simulink model "model"  (R2022b)
settings: Solver=VariableStepAuto  StartTime=0.0  StopTime=15  RelTol=1e-3
libraries: neural x114, simulink x4
(part 4 of 4)

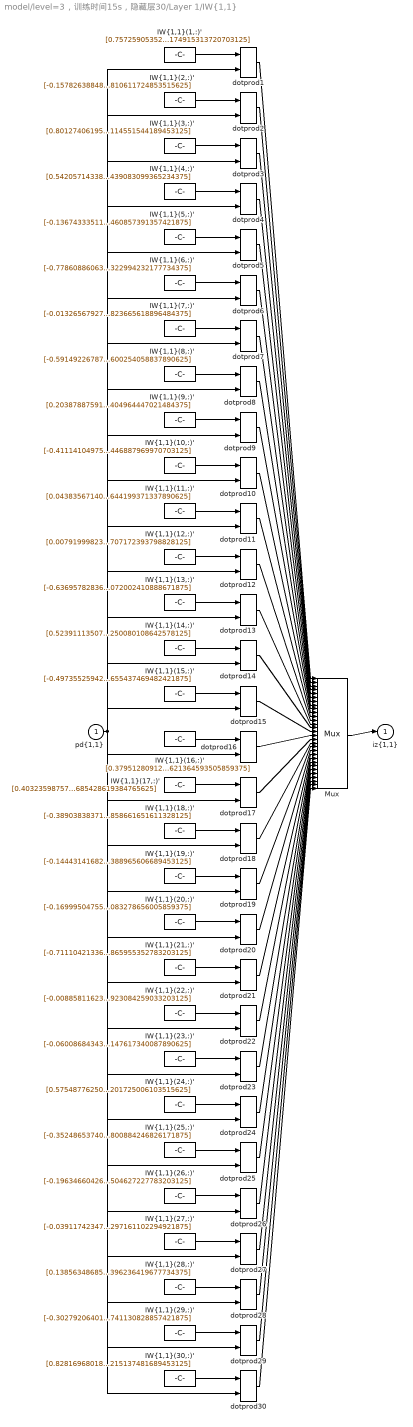
== system model/level=3，训练时间15s，隐藏层30/Layer 1/IW{1,1} ==
  "pd{1,1}" : Inport  PortDimensions=12
      mask Display: e = 0.06;c1 = [120 230 180]/255;c2 = ([120 230 180]+0)/(256+128);c3 = ([120 230 180]+128)/(256+128);patch([0 1 1 0],[0 0 1 1],c1);patch([0 1 1 1-e 1-e 0+e],[0 0 1 1-e 0+e 0+e],c2);patch([0 0 1 1-e 0+e 0+e],[0 1 1 1-e 1-e 0+e],c3);plot([0 1 1 0 0],[0 0 1 1 0]);
  "IW{1,1}(1,:)'" : Constant  Value=[0.75725905352932321168424323332146741449832916259765625;0.395079353687091294755617809641989879310131072998046875;0.284174770009599508835407277729245834052562713623046875;-0.480625127186739498075240817343001253902912139892578125;1.5532866213137079824946340522728860378265380859375;-0.2164618951796444534796393099895794875919818878173828125;1.2456775953176404403421884126146323978900909423828125;-1.10858492845372236246248576208017766475677490234375;0.639442817441132405065218335948884487152099609375;0.293978171890306894109556878902367316186428070068359375;-0.94941996422992291915221585441031493246555328369140625;0.92768764030551065236096519583952613174915313720703125]
      mask Display: e = 0.06;c1 = [120 150 230]/255;c2 = ([120 150 230]+0)/383;c3 = ([120 150 230]+128)/383;patch([0 1 1 0],[0 0 1 1],c1);patch([0 1 1 1-e 1-e 0+e],[0 0 1 1-e 0+e 0+e],c2);patch([0 0 1 1-e 0+e 0+e],[0 1 1 1-e 1-e 0+e],c3);plot([0 1 1 0 0],[0 0 1 1 0]);disp('Weights');
  "IW{1,1}(10,:)'" : Constant  Value=[-0.41114104975904297578637169863213784992694854736328125;0.638123539358462554815787370898760855197906494140625;0.8892656713827828962593002870562486350536346435546875;-0.2296787045340132060733395746865426190197467803955078125;-0.101513006637653280250788156990893185138702392578125;0.1570479389804073921954596926298108883202075958251953125;-0.5212086340938679729362092984956689178943634033203125;0.59304447094252032979255773170734755694866180419921875;0.893787792975378803106423220015130937099456787109375;0.2422359635921390308421763393198489211499691009521484375;0.393771951328514335788355538170435465872287750244140625;-0.0501811485120902400769438145289313979446887969970703125]
      mask Display: e = 0.06;c1 = [120 150 230]/255;c2 = ([120 150 230]+0)/383;c3 = ([120 150 230]+128)/383;patch([0 1 1 0],[0 0 1 1],c1);patch([0 1 1 1-e 1-e 0+e],[0 0 1 1-e 0+e 0+e],c2);patch([0 0 1 1-e 0+e 0+e],[0 1 1 1-e 1-e 0+e],c3);plot([0 1 1 0 0],[0 0 1 1 0]);disp('Weights');
  "IW{1,1}(11,:)'" : Constant  Value=[0.0438356714023393212453783007731544785201549530029296875;0.000584453236434134826282615904347039759159088134765625;0.0234071241969575731534103368858268368057906627655029296875;-0.0146965389691917636127982405014336109161376953125;0.012973200671017141860641430639589088968932628631591796875;-0.0796343916408829011199799197129323147237300872802734375;-0.92626778833588374606478055284242145717144012451171875;0.55553594240003401072414135342114605009555816650390625;0.3147831513142638204527656853315420448780059814453125;0.70814607465412660047832105192355811595916748046875;1.113472027689847099196640556328929960727691650390625;-0.486007529758314016365972065614187158644199371337890625]
      mask Display: e = 0.06;c1 = [120 150 230]/255;c2 = ([120 150 230]+0)/383;c3 = ([120 150 230]+128)/383;patch([0 1 1 0],[0 0 1 1],c1);patch([0 1 1 1-e 1-e 0+e],[0 0 1 1-e 0+e 0+e],c2);patch([0 0 1 1-e 0+e 0+e],[0 1 1 1-e 1-e 0+e],c3);plot([0 1 1 0 0],[0 0 1 1 0]);disp('Weights');
  "IW{1,1}(12,:)'" : Constant  Value=[0.00791999823281246649597786557706058374606072902679443359375;-0.000416308322128628783588555339889580864110030233860015869140625;0.007136286944569004107863374741782536148093640804290771484375;-0.004813165301803152239246141874673412530682981014251708984375;0.004455198856121612462077852256925325491465628147125244140625;-0.0158514264036779990718617483480556984432041645050048828125;0.76581982923121127981858080602250993251800537109375;1.082796206543517048004332536947913467884063720703125;1.0764809157713461917893482677754946053028106689453125;0.75575388653398001270744543944601900875568389892578125;-0.694644687537094629448120031156577169895172119140625;-0.7383832671373753431254272072692401707172393798828125]
      mask Display: e = 0.06;c1 = [120 150 230]/255;c2 = ([120 150 230]+0)/383;c3 = ([120 150 230]+128)/383;patch([0 1 1 0],[0 0 1 1],c1);patch([0 1 1 1-e 1-e 0+e],[0 0 1 1-e 0+e 0+e],c2);patch([0 0 1 1-e 0+e 0+e],[0 1 1 1-e 1-e 0+e],c3);plot([0 1 1 0 0],[0 0 1 1 0]);disp('Weights');
  "IW{1,1}(13,:)'" : Constant  Value=[-0.63695782836304826179940619113040156662464141845703125;0.629096052803664207431211252696812152862548828125;0.323311497459243757379709904853370971977710723876953125;-0.10905608847097224278765992266926332376897335052490234375;0.00182196457625318874833098004017983839730732142925262451171875;-0.40021595696852230172879671954433433711528778076171875;-0.58507556697968521319808132830075919628143310546875;-0.1289161268611479782553175255088717676699161529541015625;0.70346509838735793440633869977318681776523590087890625;0.758628536034963385503715471713803708553314208984375;1.0820696215042822085905527274007908999919891357421875;0.66331696609620649507377265763352625072002410888671875]
      mask Display: e = 0.06;c1 = [120 150 230]/255;c2 = ([120 150 230]+0)/383;c3 = ([120 150 230]+128)/383;patch([0 1 1 0],[0 0 1 1],c1);patch([0 1 1 1-e 1-e 0+e],[0 0 1 1-e 0+e 0+e],c2);patch([0 0 1 1-e 0+e 0+e],[0 1 1 1-e 1-e 0+e],c3);plot([0 1 1 0 0],[0 0 1 1 0]);disp('Weights');
  "IW{1,1}(14,:)'" : Constant  Value=[0.52391113507237629942636658597621135413646697998046875;0.748442776635961148912201679195277392864227294921875;-0.5994868462670253084212390604079701006412506103515625;-0.407014205676378637566159568450530059635639190673828125;0.6801681371389649566339130615233443677425384521484375;-0.1601777419913940903040128205248038284480571746826171875;0.591124691698642124038087786175310611724853515625;-0.60466411573088463260461367099196650087833404541015625;-0.1698340507383852282519143273020745255053043365478515625;0.322498129489360685351329038894618861377239227294921875;-0.0207917527819724036464155147996279993094503879547119140625;0.45280346894891909670377572183497250080108642578125]
      mask Display: e = 0.06;c1 = [120 150 230]/255;c2 = ([120 150 230]+0)/383;c3 = ([120 150 230]+128)/383;patch([0 1 1 0],[0 0 1 1],c1);patch([0 1 1 1-e 1-e 0+e],[0 0 1 1-e 0+e 0+e],c2);patch([0 0 1 1-e 0+e 0+e],[0 1 1 1-e 1-e 0+e],c3);plot([0 1 1 0 0],[0 0 1 1 0]);disp('Weights');
  "IW{1,1}(15,:)'" : Constant  Value=[-0.4973552594221628542214830304146744310855865478515625;-0.57340079597389592702683103198069147765636444091796875;0.2404892307980655286048232710527372546494007110595703125;0.14602880061020651059067176902317441999912261962890625;-0.4128068227448673521706723477109335362911224365234375;-0.449657532232850043474314816194237209856510162353515625;-0.437774623382925665016074390223366208374500274658203125;-0.0506924454175674277234264764047111384570598602294921875;0.03919016699132422953955057209896040149033069610595703125;-0.318569485200799917823388796023209579288959503173828125;-1.0445535535771595103682329863659106194972991943359375;1.5582165788630042424500743436510674655437469482421875]
      mask Display: e = 0.06;c1 = [120 150 230]/255;c2 = ([120 150 230]+0)/383;c3 = ([120 150 230]+128)/383;patch([0 1 1 0],[0 0 1 1],c1);patch([0 1 1 1-e 1-e 0+e],[0 0 1 1-e 0+e 0+e],c2);patch([0 0 1 1-e 0+e 0+e],[0 1 1 1-e 1-e 0+e],c3);plot([0 1 1 0 0],[0 0 1 1 0]);disp('Weights');
  "IW{1,1}(16,:)'" : Constant  Value=[0.379512809123591920990037351657520048320293426513671875;0.65302219172945097369620270910672843456268310546875;0.2093694388414068241477394849425763823091983795166015625;0.53901943330297819034768735946272499859333038330078125;0.33835271552903611880225298591540195047855377197265625;0.474312833179603376976274375920183956623077392578125;0.2112993037316006350589958628916065208613872528076171875;-0.24506554704123661991843619034625589847564697265625;0.54971876255830476321051492050173692405223846435546875;1.2430077042784175578304939335794188082218170166015625;0.4314133185581263685293151866062544286251068115234375;0.7864615366629035264622871181927621364593505859375]
      mask Display: e = 0.06;c1 = [120 150 230]/255;c2 = ([120 150 230]+0)/383;c3 = ([120 150 230]+128)/383;patch([0 1 1 0],[0 0 1 1],c1);patch([0 1 1 1-e 1-e 0+e],[0 0 1 1-e 0+e 0+e],c2);patch([0 0 1 1-e 0+e 0+e],[0 1 1 1-e 1-e 0+e],c3);plot([0 1 1 0 0],[0 0 1 1 0]);disp('Weights');
  "IW{1,1}(17,:)'" : Constant  Value=[0.403235987579470656072544443304650485515594482421875;-0.1362114449718113406984087987439124844968318939208984375;-0.1822965898937449480410322166790137998759746551513671875;-0.489926907426365965125825141512905247509479522705078125;-0.32566431987358368527196716968319378793239593505859375;-0.1290782481439954054724950083254952915012836456298828125;-0.98752010009051549577208106711623258888721466064453125;-0.155169136490018344520791515606106258928775787353515625;0.3678391748322893395339860944659449160099029541015625;-0.51093268181998385824016395417856983840465545654296875;-0.56491649164861390541858554570353589951992034912109375;-0.488184828165648898590234239236451685428619384765625]
      mask Display: e = 0.06;c1 = [120 150 230]/255;c2 = ([120 150 230]+0)/383;c3 = ([120 150 230]+128)/383;patch([0 1 1 0],[0 0 1 1],c1);patch([0 1 1 1-e 1-e 0+e],[0 0 1 1-e 0+e 0+e],c2);patch([0 0 1 1-e 0+e 0+e],[0 1 1 1-e 1-e 0+e],c3);plot([0 1 1 0 0],[0 0 1 1 0]);disp('Weights');
  "IW{1,1}(18,:)'" : Constant  Value=[-0.389038383711070634429773917872807942330837249755859375;0.420319497494296978601369119132868945598602294921875;-0.351918184281379831102043453938676975667476654052734375;0.04480775966626733552988781639214721508324146270751953125;0.1814472958334386876178001557491370476782321929931640625;-0.21879895422863615550568283651955425739288330078125;-0.358468282492263312644098505188594572246074676513671875;0.196359806412406523445923767212661914527416229248046875;0.6642308737386832806492975578294135630130767822265625;0.1549977942349778647912472706593689508736133575439453125;-0.7313716204282820765314454547478817403316497802734375;-0.63985926564271977667885948903858661651611328125]
      mask Display: e = 0.06;c1 = [120 150 230]/255;c2 = ([120 150 230]+0)/383;c3 = ([120 150 230]+128)/383;patch([0 1 1 0],[0 0 1 1],c1);patch([0 1 1 1-e 1-e 0+e],[0 0 1 1-e 0+e 0+e],c2);patch([0 0 1 1-e 0+e 0+e],[0 1 1 1-e 1-e 0+e],c3);plot([0 1 1 0 0],[0 0 1 1 0]);disp('Weights');
  "IW{1,1}(19,:)'" : Constant  Value=[-0.144431416823362857027035488499677740037441253662109375;-0.999290810935264062209171243011951446533203125;-0.6064844945590530667089979033335112035274505615234375;0.307419146554513245117590258814743719995021820068359375;0.51981343569719717923049984165118075907230377197265625;-1.022888772059110440437734723673202097415924072265625;0.2678751539195631803380592828034423291683197021484375;0.08165050161507102222113729794727987609803676605224609375;0.5316342490032222034557207734906114637851715087890625;-0.079997224310751458009605130428099073469638824462890625;-0.99517161158581834978775759736890904605388641357421875;0.07310073594289434595339116640388965606689453125]
      mask Display: e = 0.06;c1 = [120 150 230]/255;c2 = ([120 150 230]+0)/383;c3 = ([120 150 230]+128)/383;patch([0 1 1 0],[0 0 1 1],c1);patch([0 1 1 1-e 1-e 0+e],[0 0 1 1-e 0+e 0+e],c2);patch([0 0 1 1-e 0+e 0+e],[0 1 1 1-e 1-e 0+e],c3);plot([0 1 1 0 0],[0 0 1 1 0]);disp('Weights');
  "IW{1,1}(2,:)'" : Constant  Value=[-0.1578263884876335010343240128349862061440944671630859375;-0.458760873909689281813228944884031079709529876708984375;-0.305984546669152146503023459445103071630001068115234375;0.58581045035913437146746218786574900150299072265625;-0.047317706603537811049786654393756180070340633392333984375;0.42130501846705092905409628656343556940555572509765625;-0.57844534526135105156896543121547438204288482666015625;0.61224458343678289651279555982910096645355224609375;-0.9387301596170674056196503443061374127864837646484375;-0.044427698494935496942304098411113955080509185791015625;0.32438244619906420052046769342268817126750946044921875;-0.2192552159109796561242688994752825237810611724853515625]
      mask Display: e = 0.06;c1 = [120 150 230]/255;c2 = ([120 150 230]+0)/383;c3 = ([120 150 230]+128)/383;patch([0 1 1 0],[0 0 1 1],c1);patch([0 1 1 1-e 1-e 0+e],[0 0 1 1-e 0+e 0+e],c2);patch([0 0 1 1-e 0+e 0+e],[0 1 1 1-e 1-e 0+e],c3);plot([0 1 1 0 0],[0 0 1 1 0]);disp('Weights');
  "IW{1,1}(20,:)'" : Constant  Value=[-0.16999504755105177000729099745512939989566802978515625;-0.2307373712636667517639210700508556328713893890380859375;0.0887272338162874152356351942216861061751842498779296875;-0.30921237886105645831236188314505852758884429931640625;-0.085253712142476512081401551768067292869091033935546875;0.30098321919776793720302521251142024993896484375;1.0702575958242466214187516015954315662384033203125;0.31550484693018121529206609920947812497615814208984375;0.3615258196366675225164044604753144085407257080078125;-0.00158854198173050890734170348395082328352145850658416748046875;-0.423955871671502670938735946037922985851764678955078125;0.83912806509913406838307992074987851083278656005859375]
      mask Display: e = 0.06;c1 = [120 150 230]/255;c2 = ([120 150 230]+0)/383;c3 = ([120 150 230]+128)/383;patch([0 1 1 0],[0 0 1 1],c1);patch([0 1 1 1-e 1-e 0+e],[0 0 1 1-e 0+e 0+e],c2);patch([0 0 1 1-e 0+e 0+e],[0 1 1 1-e 1-e 0+e],c3);plot([0 1 1 0 0],[0 0 1 1 0]);disp('Weights');
  "IW{1,1}(21,:)'" : Constant  Value=[-0.7111042133619023264401448614080436527729034423828125;-0.6247844908542052877464811899699270725250244140625;-0.411286070103796086439018608871265314519405364990234375;0.50546004210985107096831825401750393211841583251953125;-0.017630168364032729189094794719494529999792575836181640625;0.465225631858145416419603179747355170547962188720703125;-0.489030347200887283154457918499247170984745025634765625;0.34997890668509945566455598964239470660686492919921875;1.2310428148694978478516759423655457794666290283203125;-0.236218929215159134660240169978351332247257232666015625;0.6064418661417680933567453394061885774135589599609375;0.539387507602196780709391532582230865955352783203125]
      mask Display: e = 0.06;c1 = [120 150 230]/255;c2 = ([120 150 230]+0)/383;c3 = ([120 150 230]+128)/383;patch([0 1 1 0],[0 0 1 1],c1);patch([0 1 1 1-e 1-e 0+e],[0 0 1 1-e 0+e 0+e],c2);patch([0 0 1 1-e 0+e 0+e],[0 1 1 1-e 1-e 0+e],c3);plot([0 1 1 0 0],[0 0 1 1 0]);disp('Weights');
  "IW{1,1}(22,:)'" : Constant  Value=[-0.00885811623799481924479426453444830258376896381378173828125;0.001129260518233908029694934072040268802084028720855712890625;-0.00783442931556284187510907912610491621308028697967529296875;0.0064317418415292711142416948177924496121704578399658203125;-0.005060795156085261779776995894053470692597329616546630859375;0.0202300155601852875431045930554319056682288646697998046875;0.1497182692598838238406955269965692423284053802490234375;0.62596589744369257601874778629280626773834228515625;-0.498198984154921309386310213085380382835865020751953125;-1.032780371682340270211852839565835893154144287109375;-0.01657765371532306242219334535548114217817783355712890625;0.43974659987180342302082181049627251923084259033203125]
      mask Display: e = 0.06;c1 = [120 150 230]/255;c2 = ([120 150 230]+0)/383;c3 = ([120 150 230]+128)/383;patch([0 1 1 0],[0 0 1 1],c1);patch([0 1 1 1-e 1-e 0+e],[0 0 1 1-e 0+e 0+e],c2);patch([0 0 1 1-e 0+e 0+e],[0 1 1 1-e 1-e 0+e],c3);plot([0 1 1 0 0],[0 0 1 1 0]);disp('Weights');
  "IW{1,1}(23,:)'" : Constant  Value=[-0.06008684343657157145290881317123421467840671539306640625;0.01367215496164737344175765798581778653897345066070556640625;-0.038969270528510270568123274870231398381292819976806640625;0.022194456059804433534221601576064131222665309906005859375;-0.01341113093208178529136542778132934472523629665374755859375;0.09922945233834022660257545567219494841992855072021484375;0.65314267254930225004017074752482585608959197998046875;-0.45144024693216289190189627333893440663814544677734375;-0.94194454619317913302012357235071249306201934814453125;-0.2252271298497275087147073691085097379982471466064453125;-0.205636323968237999526564863117528147995471954345703125;-0.344140829990361718504487953396164812147617340087890625]
      mask Display: e = 0.06;c1 = [120 150 230]/255;c2 = ([120 150 230]+0)/383;c3 = ([120 150 230]+128)/383;patch([0 1 1 0],[0 0 1 1],c1);patch([0 1 1 1-e 1-e 0+e],[0 0 1 1-e 0+e 0+e],c2);patch([0 0 1 1-e 0+e 0+e],[0 1 1 1-e 1-e 0+e],c3);plot([0 1 1 0 0],[0 0 1 1 0]);disp('Weights');
  "IW{1,1}(24,:)'" : Constant  Value=[0.57548776250792565978287029793136753141880035400390625;-0.45795778096452643968206075442139990627765655517578125;-0.38607748218673354489993698734906502068042755126953125;0.4916252004689363186429318375303409993648529052734375;0.2406619633258665624797600912643247283995151519775390625;-0.8457958795838391719001947421929799020290374755859375;0.372315286864318528703421407044515945017337799072265625;0.72529018681633028453603628804557956755161285400390625;0.35433543342820394972392250565462745726108551025390625;-0.41379597149052071980435130171827040612697601318359375;-0.1366403163625886374443751947183045558631420135498046875;-1.3857644267861051190493526519276201725006103515625]
      mask Display: e = 0.06;c1 = [120 150 230]/255;c2 = ([120 150 230]+0)/383;c3 = ([120 150 230]+128)/383;patch([0 1 1 0],[0 0 1 1],c1);patch([0 1 1 1-e 1-e 0+e],[0 0 1 1-e 0+e 0+e],c2);patch([0 0 1 1-e 0+e 0+e],[0 1 1 1-e 1-e 0+e],c3);plot([0 1 1 0 0],[0 0 1 1 0]);disp('Weights');
  "IW{1,1}(25,:)'" : Constant  Value=[-0.352486537409815336996388168699922971427440643310546875;0.414043250901561632471015172995976172387599945068359375;-0.68290105169643278149038678748183883726596832275390625;-0.96276684869885087447727300968836061656475067138671875;0.5424616924357665848077658665715716779232025146484375;0.1577350356187188495926676523595233447849750518798828125;0.418964763852672394950360512666520662605762481689453125;0.457891452988993197248390742970514111220836639404296875;0.08332747072123615483807412829264649190008640289306640625;0.65158691952563863036829161501373164355754852294921875;-0.76207838543505646011766430092393420636653900146484375;-1.0240547489832934058284763523261062800884246826171875]
      mask Display: e = 0.06;c1 = [120 150 230]/255;c2 = ([120 150 230]+0)/383;c3 = ([120 150 230]+128)/383;patch([0 1 1 0],[0 0 1 1],c1);patch([0 1 1 1-e 1-e 0+e],[0 0 1 1-e 0+e 0+e],c2);patch([0 0 1 1-e 0+e 0+e],[0 1 1 1-e 1-e 0+e],c3);plot([0 1 1 0 0],[0 0 1 1 0]);disp('Weights');
  "IW{1,1}(26,:)'" : Constant  Value=[-0.1963466042652797505230211072557722218334674835205078125;-0.27192840713707522315445430649560876190662384033203125;0.182210292232644344156966553782694973051548004150390625;-0.447224059368448223494851845316588878631591796875;0.1576605364208199799858078904435387812554836273193359375;0.78926919129368589000961264900979585945606231689453125;-1.2972634275407397552726251888088881969451904296875;-0.04020699212536023303687926500060711987316608428955078125;0.487034869518653767972438117794808931648731231689453125;0.6254254757920250096248082627425901591777801513671875;-0.26065496508075458592657014378346502780914306640625;-1.0041097040721507216431973574799485504627227783203125]
      mask Display: e = 0.06;c1 = [120 150 230]/255;c2 = ([120 150 230]+0)/383;c3 = ([120 150 230]+128)/383;patch([0 1 1 0],[0 0 1 1],c1);patch([0 1 1 1-e 1-e 0+e],[0 0 1 1-e 0+e 0+e],c2);patch([0 0 1 1-e 0+e 0+e],[0 1 1 1-e 1-e 0+e],c3);plot([0 1 1 0 0],[0 0 1 1 0]);disp('Weights');
  "IW{1,1}(27,:)'" : Constant  Value=[-0.03911742347526304952598508180017233826220035552978515625;0.494928256667255705991692593670450150966644287109375;-0.461046038716595718565116612808196805417537689208984375;-0.475821016979017408221608320673112757503986358642578125;0.1715992837547896388006307688556262291967868804931640625;0.441321179942003372076442246907390654087066650390625;0.07770246050736133447411901897794450633227825164794921875;-0.7399663724277554255337463473551906645298004150390625;-0.054265638891030233692536199896494508720934391021728515625;-0.84771877074509627281173607116215862333774566650390625;0.491481003922895232083334349226788617670536041259765625;0.362234471234642974035722318149055354297161102294921875]
      mask Display: e = 0.06;c1 = [120 150 230]/255;c2 = ([120 150 230]+0)/383;c3 = ([120 150 230]+128)/383;patch([0 1 1 0],[0 0 1 1],c1);patch([0 1 1 1-e 1-e 0+e],[0 0 1 1-e 0+e 0+e],c2);patch([0 0 1 1-e 0+e 0+e],[0 1 1 1-e 1-e 0+e],c3);plot([0 1 1 0 0],[0 0 1 1 0]);disp('Weights');
  "IW{1,1}(28,:)'" : Constant  Value=[0.1385634868509460215779682812353712506592273712158203125;0.1279689227168545329060833637413452379405498504638671875;-0.11494143852620981871570648991109919734299182891845703125;0.20340717598419566503054056738619692623615264892578125;0.08727794408846646645461220259676338173449039459228515625;-0.283290172800760908788930692026042379438877105712890625;0.160823631436447567200076491644722409546375274658203125;-0.320376770185884340857995766782551072537899017333984375;0.737629304081023118300208807340823113918304443359375;0.63998442620449991213860130301327444612979888916015625;-0.92223956712347021635878263623453676700592041015625;-0.49126791669202185541820426806225441396236419677734375]
      mask Display: e = 0.06;c1 = [120 150 230]/255;c2 = ([120 150 230]+0)/383;c3 = ([120 150 230]+128)/383;patch([0 1 1 0],[0 0 1 1],c1);patch([0 1 1 1-e 1-e 0+e],[0 0 1 1-e 0+e 0+e],c2);patch([0 0 1 1-e 0+e 0+e],[0 1 1 1-e 1-e 0+e],c3);plot([0 1 1 0 0],[0 0 1 1 0]);disp('Weights');
  "IW{1,1}(29,:)'" : Constant  Value=[-0.30279206401474556553665706815081648528575897216796875;-0.412469215746285422508066176305874250829219818115234375;-0.432449526865937350361690505451406352221965789794921875;-0.56925500452449007138255865356768481433391571044921875;-0.059863877680234288403138265266534290276467800140380859375;0.58350248883230182439518785031395964324474334716796875;-0.669606012141286566219378073583357036113739013671875;-0.97190522552113300935872075569932349026203155517578125;-0.63078228616375719983722092365496791899204254150390625;0.70291498121659945486072729181614704430103302001953125;-0.614409800146754836447371417307294905185699462890625;0.125911678355542289153845558757893741130828857421875]
      mask Display: e = 0.06;c1 = [120 150 230]/255;c2 = ([120 150 230]+0)/383;c3 = ([120 150 230]+128)/383;patch([0 1 1 0],[0 0 1 1],c1);patch([0 1 1 1-e 1-e 0+e],[0 0 1 1-e 0+e 0+e],c2);patch([0 0 1 1-e 0+e 0+e],[0 1 1 1-e 1-e 0+e],c3);plot([0 1 1 0 0],[0 0 1 1 0]);disp('Weights');
  "IW{1,1}(3,:)'" : Constant  Value=[0.8012740619552223275690039372420869767665863037109375;-0.7633715123897300003363852738402783870697021484375;-0.465703691458938251468424596168915741145610809326171875;0.03666851099753165588168712929473258554935455322265625;-0.2460643798862774678237741454722709022462368011474609375;-0.162877941160530503861281204081024043262004852294921875;0.545551433681740416403727067518047988414764404296875;0.94833875724121974304381410547648556530475616455078125;0.52080467915547845603185805885004810988903045654296875;0.2174677890345051156639755163269001059234142303466796875;-1.068422894633431763367070743697695434093475341796875;0.334523901695165382097485462509212084114551544189453125]
      mask Display: e = 0.06;c1 = [120 150 230]/255;c2 = ([120 150 230]+0)/383;c3 = ([120 150 230]+128)/383;patch([0 1 1 0],[0 0 1 1],c1);patch([0 1 1 1-e 1-e 0+e],[0 0 1 1-e 0+e 0+e],c2);patch([0 0 1 1-e 0+e 0+e],[0 1 1 1-e 1-e 0+e],c3);plot([0 1 1 0 0],[0 0 1 1 0]);disp('Weights');
  "IW{1,1}(30,:)'" : Constant  Value=[0.82816968018509573568053383496589958667755126953125;0.9201804860082936077247950379387475550174713134765625;0.0955833140605594488992124979631626047194004058837890625;0.572857804385419999704254223615862429141998291015625;0.5228942181369493624742972315289080142974853515625;0.7683928307468963492254943048465065658092498779296875;0.583383677465624916891329121426679193973541259765625;0.288500493038154781633153334041708149015903472900390625;0.482505378597943235252643034982611425220966339111328125;0.0061240261079962728107961567047823336906731128692626953125;0.9410942585011101702008318170555867254734039306640625;0.148252366927580869759850656919297762215137481689453125]
      mask Display: e = 0.06;c1 = [120 150 230]/255;c2 = ([120 150 230]+0)/383;c3 = ([120 150 230]+128)/383;patch([0 1 1 0],[0 0 1 1],c1);patch([0 1 1 1-e 1-e 0+e],[0 0 1 1-e 0+e 0+e],c2);patch([0 0 1 1-e 0+e 0+e],[0 1 1 1-e 1-e 0+e],c3);plot([0 1 1 0 0],[0 0 1 1 0]);disp('Weights');
  "IW{1,1}(4,:)'" : Constant  Value=[0.5420571433834135977036794429295696318149566650390625;-0.1474756847674350279664423624126357026398181915283203125;-0.365439776403620630862434381924686022102832794189453125;0.7077497085807333832008225726895034313201904296875;1.0487685096710299692546186633990146219730377197265625;-0.35569914837861171807986693238490261137485504150390625;-0.552399027313476675971060103620402514934539794921875;-0.2147081738626088476262765425417455844581127166748046875;0.59383018589869662751112855403334833681583404541015625;0.85026968267060476502905430606915615499019622802734375;-0.0192523512445413429172713648540593567304313182830810546875;0.0287311566380798986963807095662559731863439083099365234375]
      mask Display: e = 0.06;c1 = [120 150 230]/255;c2 = ([120 150 230]+0)/383;c3 = ([120 150 230]+128)/383;patch([0 1 1 0],[0 0 1 1],c1);patch([0 1 1 1-e 1-e 0+e],[0 0 1 1-e 0+e 0+e],c2);patch([0 0 1 1-e 0+e 0+e],[0 1 1 1-e 1-e 0+e],c3);plot([0 1 1 0 0],[0 0 1 1 0]);disp('Weights');
  "IW{1,1}(5,:)'" : Constant  Value=[-0.1367433351147859521557137441050144843757152557373046875;-0.060410553566593007401852588600377202965319156646728515625;0.10997569628914076467207650011914665810763835906982421875;-0.004579366895770255359299216735280424472875893115997314453125;0.290226317818353229949224214578862302005290985107421875;0.3481346428669691572821420777472667396068572998046875;0.496980705700768410348899806194822303950786590576171875;-0.4878505757218436489353052820661105215549468994140625;-0.292932542648377147731508785000187344849109649658203125;-0.64064664844808183463698014747933484613895416259765625;-1.1368564158628868820954949114820919930934906005859375;0.52022106413102242594703739086980931460857391357421875]
      mask Display: e = 0.06;c1 = [120 150 230]/255;c2 = ([120 150 230]+0)/383;c3 = ([120 150 230]+128)/383;patch([0 1 1 0],[0 0 1 1],c1);patch([0 1 1 1-e 1-e 0+e],[0 0 1 1-e 0+e 0+e],c2);patch([0 0 1 1-e 0+e 0+e],[0 1 1 1-e 1-e 0+e],c3);plot([0 1 1 0 0],[0 0 1 1 0]);disp('Weights');
  "IW{1,1}(6,:)'" : Constant  Value=[-0.7786088606380554555386197534971870481967926025390625;1.0631936368359100608671496956958435475826263427734375;0.7410329806340187897006899220286868512630462646484375;0.48671035274339813359034678796888329088687896728515625;-0.16755322222335333748333141556940972805023193359375;-1.052994665323438550075252351234667003154754638671875;0.55960633469295950614963430780335329473018646240234375;1.0334851014872141750089440392912365496158599853515625;-0.18471697837201939140783224502229131758213043212890625;0.060399284747913152548992599122357205487787723541259765625;-0.33699098710674346701665626824251376092433929443359375;-0.231368893896155947143000730648054741322994232177734375]
      mask Display: e = 0.06;c1 = [120 150 230]/255;c2 = ([120 150 230]+0)/383;c3 = ([120 150 230]+128)/383;patch([0 1 1 0],[0 0 1 1],c1);patch([0 1 1 1-e 1-e 0+e],[0 0 1 1-e 0+e 0+e],c2);patch([0 0 1 1-e 0+e 0+e],[0 1 1 1-e 1-e 0+e],c3);plot([0 1 1 0 0],[0 0 1 1 0]);disp('Weights');
  "IW{1,1}(7,:)'" : Constant  Value=[-0.0132656792799620941447624744569111499004065990447998046875;-0.00109241586046383300744044841934510259306989610195159912109375;-0.0161138187616071508478921003870709682814776897430419921875;0.012457151836826003965530418327034567482769489288330078125;-0.00814316138631742368614307991947498521767556667327880859375;0.030624545708644874963955118118974496610462665557861328125;-0.55159842387257762563734786454006098210811614990234375;0.35132025843639447248989426952903158962726593017578125;0.6901610288367854284530267250374890863895416259765625;0.08295849322685887317074815427986322902143001556396484375;-0.65282286739034589562180599386920221149921417236328125;-0.430855205660852946802918950197636149823665618896484375]
      mask Display: e = 0.06;c1 = [120 150 230]/255;c2 = ([120 150 230]+0)/383;c3 = ([120 150 230]+128)/383;patch([0 1 1 0],[0 0 1 1],c1);patch([0 1 1 1-e 1-e 0+e],[0 0 1 1-e 0+e 0+e],c2);patch([0 0 1 1-e 0+e 0+e],[0 1 1 1-e 1-e 0+e],c3);plot([0 1 1 0 0],[0 0 1 1 0]);disp('Weights');
  "IW{1,1}(8,:)'" : Constant  Value=[-0.5914922678721143967095486004836857318878173828125;0.1542183272763184564979610513546504080295562744140625;-0.4595809487012003646810853751958347856998443603515625;-0.1405069870888906724548661486551281996071338653564453125;-0.5823603127411878244146237193490378558635711669921875;0.602835725793367860347871101112104952335357666015625;-0.75253374870000400154168573862989433109760284423828125;-0.463913367975307633361836678886902518570423126220703125;0.8908048921767466321597339629079215228557586669921875;-0.5813444755329033597490706597454845905303955078125;-0.83879002630134891216329151575337164103984832763671875;0.202672827905192642905518596307956613600254058837890625]
      mask Display: e = 0.06;c1 = [120 150 230]/255;c2 = ([120 150 230]+0)/383;c3 = ([120 150 230]+128)/383;patch([0 1 1 0],[0 0 1 1],c1);patch([0 1 1 1-e 1-e 0+e],[0 0 1 1-e 0+e 0+e],c2);patch([0 0 1 1-e 0+e 0+e],[0 1 1 1-e 1-e 0+e],c3);plot([0 1 1 0 0],[0 0 1 1 0]);disp('Weights');
  "IW{1,1}(9,:)'" : Constant  Value=[0.2038788759172467102143144757064874283969402313232421875;0.9175756806186854408480257916380651295185089111328125;0.43837184921573857376841942823375575244426727294921875;0.63113247497029700827653186934185214340686798095703125;0.5098618110055361807297913401271216571331024169921875;-0.061984745820637253410634315287097706459462642669677734375;-0.67027740871008634204741838402696885168552398681640625;0.93645585298595179768454954682965762913227081298828125;-0.1298098262110914113964810212564771063625812530517578125;0.34103186031137600053853020654059946537017822265625;-0.299637042573452860860783175667165778577327728271484375;0.36984091827835940957669436102150939404964447021484375]
      mask Display: e = 0.06;c1 = [120 150 230]/255;c2 = ([120 150 230]+0)/383;c3 = ([120 150 230]+128)/383;patch([0 1 1 0],[0 0 1 1],c1);patch([0 1 1 1-e 1-e 0+e],[0 0 1 1-e 0+e 0+e],c2);patch([0 0 1 1-e 0+e 0+e],[0 1 1 1-e 1-e 0+e],c3);plot([0 1 1 0 0],[0 0 1 1 0]);disp('Weights');
  Mux : Mux  Inputs=30
      mask Display: e = 0.06;c1 = [120 150 230]/255;c2 = ([120 150 230]+0)/383;c3 = ([120 150 230]+128)/383;patch([0 1 1 0],[0 0 1 1],c1);patch([0 1 1 1-e 1-e 0+e],[0 0 1 1-e 0+e 0+e],c2);patch([0 0 1 1-e 0+e 0+e],[0 1 1 1-e 1-e 0+e],c3);plot([0 1 1 0 0],[0 0 1 1 0]);disp('Mux');
  dotprod{1..30} (30 alike) : neural/Weight Functions/dotprod
  "iz{1,1}" : Outport
      mask Display: e = 0.06;c1 = [120 230 180]/255;c2 = ([120 230 180]+0)/(256+128);c3 = ([120 230 180]+128)/(256+128);patch([0 1 1 0],[0 0 1 1],c1);patch([0 1 1 1-e 1-e 0+e],[0 0 1 1-e 0+e 0+e],c2);patch([0 0 1 1-e 0+e 0+e],[0 1 1 1-e 1-e 0+e],c3);plot([0 1 1 0 0],[0 0 1 1 0]);
  wires:
  "IW{1,1}(1,:)'"/1 -> dotprod1/1
  "pd{1,1}"/1 -> dotprod1/2, dotprod2/2, dotprod3/2, dotprod4/2, dotprod5/2, dotprod6/2, dotprod7/2, dotprod8/2, dotprod9/2, dotprod10/2, dotprod11/2, dotprod12/2, dotprod13/2, dotprod14/2, dotprod15/2, dotprod16/2, dotprod17/2, dotprod18/2, dotprod19/2, dotprod20/2, dotprod21/2, dotprod22/2, dotprod23/2, dotprod24/2, dotprod25/2, dotprod26/2, dotprod27/2, dotprod28/2, dotprod29/2, dotprod30/2
  dotprod1/1 -> Mux/1
  "IW{1,1}(2,:)'"/1 -> dotprod2/1
  dotprod2/1 -> Mux/2
  "IW{1,1}(3,:)'"/1 -> dotprod3/1
  dotprod3/1 -> Mux/3
  "IW{1,1}(4,:)'"/1 -> dotprod4/1
  dotprod4/1 -> Mux/4
  "IW{1,1}(5,:)'"/1 -> dotprod5/1
  dotprod5/1 -> Mux/5
  "IW{1,1}(6,:)'"/1 -> dotprod6/1
  dotprod6/1 -> Mux/6
  "IW{1,1}(7,:)'"/1 -> dotprod7/1
  dotprod7/1 -> Mux/7
  "IW{1,1}(8,:)'"/1 -> dotprod8/1
  dotprod8/1 -> Mux/8
  "IW{1,1}(9,:)'"/1 -> dotprod9/1
  dotprod9/1 -> Mux/9
  "IW{1,1}(10,:)'"/1 -> dotprod10/1
  dotprod10/1 -> Mux/10
  "IW{1,1}(11,:)'"/1 -> dotprod11/1
  dotprod11/1 -> Mux/11
  "IW{1,1}(12,:)'"/1 -> dotprod12/1
  dotprod12/1 -> Mux/12
  "IW{1,1}(13,:)'"/1 -> dotprod13/1
  dotprod13/1 -> Mux/13
  "IW{1,1}(14,:)'"/1 -> dotprod14/1
  dotprod14/1 -> Mux/14
  "IW{1,1}(15,:)'"/1 -> dotprod15/1
  dotprod15/1 -> Mux/15
  "IW{1,1}(16,:)'"/1 -> dotprod16/1
  dotprod16/1 -> Mux/16
  "IW{1,1}(17,:)'"/1 -> dotprod17/1
  dotprod17/1 -> Mux/17
  "IW{1,1}(18,:)'"/1 -> dotprod18/1
  dotprod18/1 -> Mux/18
  "IW{1,1}(19,:)'"/1 -> dotprod19/1
  dotprod19/1 -> Mux/19
  "IW{1,1}(20,:)'"/1 -> dotprod20/1
  dotprod20/1 -> Mux/20
  "IW{1,1}(21,:)'"/1 -> dotprod21/1
  dotprod21/1 -> Mux/21
  "IW{1,1}(22,:)'"/1 -> dotprod22/1
  dotprod22/1 -> Mux/22
  "IW{1,1}(23,:)'"/1 -> dotprod23/1
  dotprod23/1 -> Mux/23
  "IW{1,1}(24,:)'"/1 -> dotprod24/1
  dotprod24/1 -> Mux/24
  "IW{1,1}(25,:)'"/1 -> dotprod25/1
  dotprod25/1 -> Mux/25
  "IW{1,1}(26,:)'"/1 -> dotprod26/1
  dotprod26/1 -> Mux/26
  "IW{1,1}(27,:)'"/1 -> dotprod27/1
  dotprod27/1 -> Mux/27
  "IW{1,1}(28,:)'"/1 -> dotprod28/1
  dotprod28/1 -> Mux/28
  "IW{1,1}(29,:)'"/1 -> dotprod29/1
  dotprod29/1 -> Mux/29
  "IW{1,1}(30,:)'"/1 -> dotprod30/1
  dotprod30/1 -> Mux/30
  Mux/1 -> "iz{1,1}"/1

== system model/level=3，训练时间15s，隐藏层30/Layer 2/Delays 1 ==
  "p{2}" : Inport  PortDimensions=30
      mask Display: e = 0.06;c1 = [120 230 180]/255;c2 = ([120 230 180]+0)/(256+128);c3 = ([120 230 180]+128)/(256+128);patch([0 1 1 0],[0 0 1 1],c1);patch([0 1 1 1-e 1-e 0+e],[0 0 1 1-e 0+e 0+e],c2);patch([0 0 1 1-e 0+e 0+e],[0 1 1 1-e 1-e 0+e],c3);plot([0 1 1 0 0],[0 0 1 1 0]);
  mux : Mux  Inputs=1
      mask Display: e = 0.06;c1 = [120 150 230]/255;c2 = ([120 150 230]+0)/383;c3 = ([120 150 230]+128)/383;patch([0 1 1 0],[0 0 1 1],c1);patch([0 1 1 1-e 1-e 0+e],[0 0 1 1-e 0+e 0+e],c2);patch([0 0 1 1-e 0+e 0+e],[0 1 1 1-e 1-e 0+e],c3);plot([0 1 1 0 0],[0 0 1 1 0]);disp('Mux')
  "pd{2,1}" : Outport
      mask Display: e = 0.06;c1 = [120 230 180]/255;c2 = ([120 230 180]+0)/(256+128);c3 = ([120 230 180]+128)/(256+128);patch([0 1 1 0],[0 0 1 1],c1);patch([0 1 1 1-e 1-e 0+e],[0 0 1 1-e 0+e 0+e],c2);patch([0 0 1 1-e 0+e 0+e],[0 1 1 1-e 1-e 0+e],c3);plot([0 1 1 0 0],[0 0 1 1 0]);
  wires:
  "p{2}"/1 -> mux/1
  mux/1 -> "pd{2,1}"/1

== system model/level=3，训练时间15s，隐藏层30/Layer 2/LW{2,1} ==
  "ad{2,1}" : Inport  PortDimensions=30
      mask Display: e = 0.06;c1 = [120 230 180]/255;c2 = ([120 230 180]+0)/(256+128);c3 = ([120 230 180]+128)/(256+128);patch([0 1 1 0],[0 0 1 1],c1);patch([0 1 1 1-e 1-e 0+e],[0 0 1 1-e 0+e 0+e],c2);patch([0 0 1 1-e 0+e 0+e],[0 1 1 1-e 1-e 0+e],c3);plot([0 1 1 0 0],[0 0 1 1 0]);
  "IW{2,1}(1,:)'" : Constant  Value=[-4.7844812106344409750012525162077281493111513555049896240234375e-05;0.000915206025194356914513604817074110542307607829570770263671875;-0.002026035468688230402334315982670887024141848087310791015625;-0.000201429424031018670417092497615385582321323454380035400390625;-0.03186222401957954086793023407153668813407421112060546875;-0.000908337037649134732865408015101138516911305487155914306640625;-0.89625138246402380470811976920231245458126068115234375;0.000583868017048882787141395045438230226864106953144073486328125;0.000408848358632767755992121205821376861422322690486907958984375;0.00088198426340384901596369804366304379072971642017364501953125;-0.63685642908871031853124122790177352726459503173828125;0.57921875650081833253324248289573006331920623779296875;-0.00201542116492167515395816934642425621859729290008544921875;-0.0010509794897387556879275738452861332916654646396636962890625;-0.0003317780963279632591884926728909022131119854748249053955078125;-0.00103449120881452688060220257426635726005770266056060791015625;0.00729846740853702657947366105872788466513156890869140625;-0.00899375469241136225873045617618117830716073513031005859375;0.0002053833406379167538825802896695904564694501459598541259765625;-0.0175616202345620329994257957650916068814694881439208984375;0.000563903692475821948469627553635064032278023660182952880859375;-1.6746929166733846017223186208866536617279052734375;0.28892900478191918534065507628838531672954559326171875;-0.000505957277224126380187063656279633505619131028652191162109375;0.000153942745808208496412217147764067703974433243274688720703125;-0.005749260664177855036094388907486063544638454914093017578125;-0.001079274716842258154125833158332170569337904453277587890625;0.12206704643115422193044850018850411288440227508544921875;0.0027847424122643582751479574000086358864791691303253173828125;0.00109185292603294144438141888286963876453228294849395751953125]
      mask Display: e = 0.06;c1 = [120 150 230]/255;c2 = ([120 150 230]+0)/383;c3 = ([120 150 230]+128)/383;patch([0 1 1 0],[0 0 1 1],c1);patch([0 1 1 1-e 1-e 0+e],[0 0 1 1-e 0+e 0+e],c2);patch([0 0 1 1-e 0+e 0+e],[0 1 1 1-e 1-e 0+e],c3);plot([0 1 1 0 0],[0 0 1 1 0]);disp('weights');
  "IW{2,1}(2,:)'" : Constant  Value=[-8.0309161696754123691173454790970254180137999355792999267578125e-05;-0.0021584163512311581138714000616118937614373862743377685546875;0.0018506537804579129870286013925806400948204100131988525390625;-4.45460595356136318891983327805661474485532380640506744384765625e-05;0.034297060535940261660758920925218262709677219390869140625;0.000789107116596712908178357093191834792378358542919158935546875;1.0489735729475675451993765818770043551921844482421875;-0.000600077342875495974884592076392664239392615854740142822265625;-0.00018791378451835953817573854340849948130198754370212554931640625;-0.0004442146278683788292694634147750321062630973756313323974609375;0.48340752054396374237654754324466921389102935791015625;0.454678641683190332134500977190327830612659454345703125;0.00121640630370433745766067801241661072708666324615478515625;0.000528860310214136959162944950918472386547364294528961181640625;0.000626009164113518743778608044436850832425989210605621337890625;0.000474868034244286369403853509396640220074914395809173583984375;-0.0058088542236990718670153199809647048823535442352294921875;0.00857426679714448462810150175528178806416690349578857421875;-0.00011795966956031103092979173130316894457791931927204132080078125;0.01425490756266767876370149537024190067313611507415771484375;-0.0010540066692937524912843105795445808325894176959991455078125;1.8811549658009718566376022863551042973995208740234375;-0.22673004099511107067854709384846501052379608154296875;0.000670462650311319692530975800082160276360809803009033203125;-0.00017717373168387787999052129794819165908847935497760772705078125;0.00478975583192282373945491968925125547684729099273681640625;4.96852566683119055619168025206278116456815041601657867431640625e-05;-0.095369094373764784489111434595542959868907928466796875;-0.0025616605135463589755506763623316146549768745899200439453125;-0.0010369343908516602710545573273748232168145477771759033203125]
      mask Display: e = 0.06;c1 = [120 150 230]/255;c2 = ([120 150 230]+0)/383;c3 = ([120 150 230]+128)/383;patch([0 1 1 0],[0 0 1 1],c1);patch([0 1 1 1-e 1-e 0+e],[0 0 1 1-e 0+e 0+e],c2);patch([0 0 1 1-e 0+e 0+e],[0 1 1 1-e 1-e 0+e],c3);plot([0 1 1 0 0],[0 0 1 1 0]);disp('weights');
  Mux : Mux  Inputs=2
      mask Display: e = 0.06;c1 = [120 150 230]/255;c2 = ([120 150 230]+0)/383;c3 = ([120 150 230]+128)/383;patch([0 1 1 0],[0 0 1 1],c1);patch([0 1 1 1-e 1-e 0+e],[0 0 1 1-e 0+e 0+e],c2);patch([0 0 1 1-e 0+e 0+e],[0 1 1 1-e 1-e 0+e],c3);plot([0 1 1 0 0],[0 0 1 1 0]);disp('Mux');
  dotprod1 : neural/Weight Functions/dotprod
  dotprod2 : neural/Weight Functions/dotprod
  "lz{2,1}" : Outport
      mask Display: e = 0.06;c1 = [120 230 180]/255;c2 = ([120 230 180]+0)/(256+128);c3 = ([120 230 180]+128)/(256+128);patch([0 1 1 0],[0 0 1 1],c1);patch([0 1 1 1-e 1-e 0+e],[0 0 1 1-e 0+e 0+e],c2);patch([0 0 1 1-e 0+e 0+e],[0 1 1 1-e 1-e 0+e],c3);plot([0 1 1 0 0],[0 0 1 1 0]);
  wires:
  "IW{2,1}(1,:)'"/1 -> dotprod1/1
  "ad{2,1}"/1 -> dotprod1/2, dotprod2/2
  dotprod1/1 -> Mux/1
  "IW{2,1}(2,:)'"/1 -> dotprod2/1
  dotprod2/1 -> Mux/2
  Mux/1 -> "lz{2,1}"/1

== system model/延时/Subsystem4/Subsystem ==
  In1 : Inport
  Unit Delay : UnitDelay  SampleTime=-1  HasFrameUpgradeWarning=on
  Unit Delay1 : UnitDelay  SampleTime=-1  HasFrameUpgradeWarning=on
  Out1 : Outport
  Out2 : Outport  Port=2
  wires:
  Unit Delay1/1 -> Out2/1
  In1/1 -> Unit Delay/1
  Unit Delay/1 -> Out1/1, Unit Delay1/1

== system model/延时/Subsystem4/Subsystem1 ==
  In1 : Inport
  Unit Delay : UnitDelay  SampleTime=-1  HasFrameUpgradeWarning=on
  Unit Delay1 : UnitDelay  SampleTime=-1  HasFrameUpgradeWarning=on
  Out1 : Outport
  Out2 : Outport  Port=2
  wires:
  Unit Delay1/1 -> Out2/1
  In1/1 -> Unit Delay/1
  Unit Delay/1 -> Out1/1, Unit Delay1/1

== system model/延时/Subsystem4/Subsystem2 ==
  In1 : Inport
  Unit Delay : UnitDelay  SampleTime=-1  HasFrameUpgradeWarning=on
  Unit Delay1 : UnitDelay  SampleTime=-1  HasFrameUpgradeWarning=on
  Out1 : Outport
  Out2 : Outport  Port=2
  wires:
  Unit Delay1/1 -> Out2/1
  In1/1 -> Unit Delay/1
  Unit Delay/1 -> Out1/1, Unit Delay1/1

== system model/延时/Subsystem4/Subsystem3 ==
  In1 : Inport
  Unit Delay : UnitDelay  SampleTime=-1  HasFrameUpgradeWarning=on
  Unit Delay1 : UnitDelay  SampleTime=-1  HasFrameUpgradeWarning=on
  Out1 : Outport
  Out2 : Outport  Port=2
  wires:
  Unit Delay1/1 -> Out2/1
  In1/1 -> Unit Delay/1
  Unit Delay/1 -> Out1/1, Unit Delay1/1

== system model/延时1/Subsystem4/Subsystem ==
  In1 : Inport
  Unit Delay : UnitDelay  SampleTime=-1  HasFrameUpgradeWarning=on
  Unit Delay1 : UnitDelay  SampleTime=-1  HasFrameUpgradeWarning=on
  Unit Delay2 : UnitDelay  SampleTime=-1  HasFrameUpgradeWarning=on
  "tau1_{k-1}" : Outport
  "tau1_{k-2}" : Outport  Port=2
  out3 : Outport  Port=3
  wires:
  Unit Delay1/1 -> Unit Delay2/1, "tau1_{k-2}"/1
  In1/1 -> Unit Delay/1
  Unit Delay/1 -> "tau1_{k-1}"/1, Unit Delay1/1
  Unit Delay2/1 -> out3/1

== system model/延时1/Subsystem4/Subsystem1 ==
  In1 : Inport
  Unit Delay : UnitDelay  SampleTime=-1  HasFrameUpgradeWarning=on
  Unit Delay1 : UnitDelay  SampleTime=-1  HasFrameUpgradeWarning=on
  Unit Delay2 : UnitDelay  SampleTime=-1  HasFrameUpgradeWarning=on
  "tau2_{k-1}" : Outport
  "tau2_{k-2}" : Outport  Port=2
  out3 : Outport  Port=3
  wires:
  Unit Delay1/1 -> Unit Delay2/1, "tau2_{k-2}"/1
  In1/1 -> Unit Delay/1
  Unit Delay/1 -> "tau2_{k-1}"/1, Unit Delay1/1
  Unit Delay2/1 -> out3/1

== system model/延时1/Subsystem4/Subsystem2 ==
  y1 : Inport
  Unit Delay : UnitDelay  SampleTime=-1  HasFrameUpgradeWarning=on
  Unit Delay1 : UnitDelay  SampleTime=-1  HasFrameUpgradeWarning=on
  Unit Delay2 : UnitDelay  SampleTime=-1  HasFrameUpgradeWarning=on
  out1 : Outport
  out2 : Outport  Port=2
  out3 : Outport  Port=3
  wires:
  Unit Delay1/1 -> Unit Delay2/1, out2/1
  y1/1 -> Unit Delay/1
  Unit Delay/1 -> out1/1, Unit Delay1/1
  Unit Delay2/1 -> out3/1

== system model/延时1/Subsystem4/Subsystem4 ==
  y1 : Inport
  Unit Delay : UnitDelay  SampleTime=-1  HasFrameUpgradeWarning=on
  Unit Delay1 : UnitDelay  SampleTime=-1  HasFrameUpgradeWarning=on
  Unit Delay2 : UnitDelay  SampleTime=-1  HasFrameUpgradeWarning=on
  out1 : Outport
  out2 : Outport  Port=2
  out3 : Outport  Port=3
  wires:
  Unit Delay1/1 -> Unit Delay2/1, out2/1
  y1/1 -> Unit Delay/1
  Unit Delay/1 -> out1/1, Unit Delay1/1
  Unit Delay2/1 -> out3/1

== matlab function model/pytroch训练，40s，隐藏层[32,16] ==
  data: u input; y output
function y = predictWithONNX(u)
    persistent model; 
    coder.extrinsic('importONNXNetwork'); % 声明外部函数
    if isempty(model)
        % 仅当模型未加载时加载 ONNX 模型，防止重复加载消耗时间
        model = importONNXNetwork('model_level2.onnx', ...
            'OutputLayerType', 'regression', ...
            'InputDataFormats', 'BC');  % B=batch size, C=channels
    end

    y = zeros(1, 2);    % 初始化输出并调整输入格式
    u = reshape(u, [1, 8]);  % 确保输入尺寸匹配
    coder.extrinsic('predict');
    y_single = predict(model, u);  % 返回的预测结果是 single 类型
    y = double(y_single);  % 将结果转换为 double 类型
end
